simulink model "Planta_1_alternativa"  (Simulink 7.9)
settings: Solver=ode45  StartTime=0.0  StopTime=10.0  RelTol=1e-3
settings Model: Creator=Carlos  LastModifiedBy=Carlos

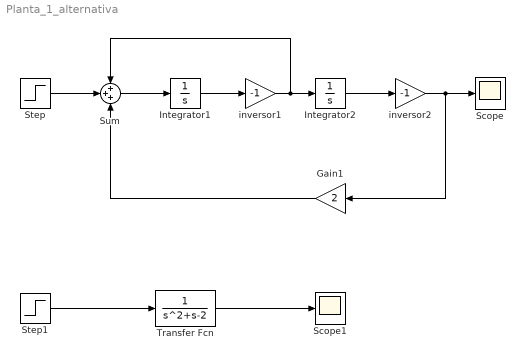
== system Planta_1_alternativa ==
  Gain1 : Gain  Gain=2
  Integrator1 : Integrator  LimitOutput=on  UpperSaturationLimit=10.5  LowerSaturationLimit=-10.5
  Integrator2 : Integrator  LimitOutput=on  UpperSaturationLimit=10.5  LowerSaturationLimit=-10.5
  Scope : Scope
  Scope1 : Scope
      settings: TimeRange=10  YMin=0  YMax=3000
  Step : Step  SampleTime=0
  Step1 : Step  SampleTime=0
  Sum : Sum  Inputs=+++
  Transfer Fcn : TransferFcn  Denominator=[1 1 -2]
  inversor1 : Gain  Gain=-1
  inversor2 : Gain  Gain=-1
  wires:
  Step1/1 -> Transfer Fcn/1
  Transfer Fcn/1 -> Scope1/1
  Sum/1 -> Integrator1/1
  Integrator1/1 -> inversor1/1
  inversor1/1 -> Integrator2/1, Sum/1
  Integrator2/1 -> inversor2/1
  inversor2/1 -> Scope/1, Gain1/1
  Step/1 -> Sum/2
  Gain1/1 -> Sum/3
